simulink model "inverter_pwmDC_test"  (R2018b)
settings: Solver=ode23tb  StartTime=0.0  StopTime=10.0  RelTol=1e-3
undefined symbols (not defined in the file): Cfmax, Lf, RLf, Tss
libraries: powerlib x8, powerlib_meascontrol x4, dspsrcs4 x3, pePowerMeasurement x2, re_lib x1, simulink x1
settings Model: Creator=samuel  LastModifiedBy=samuel

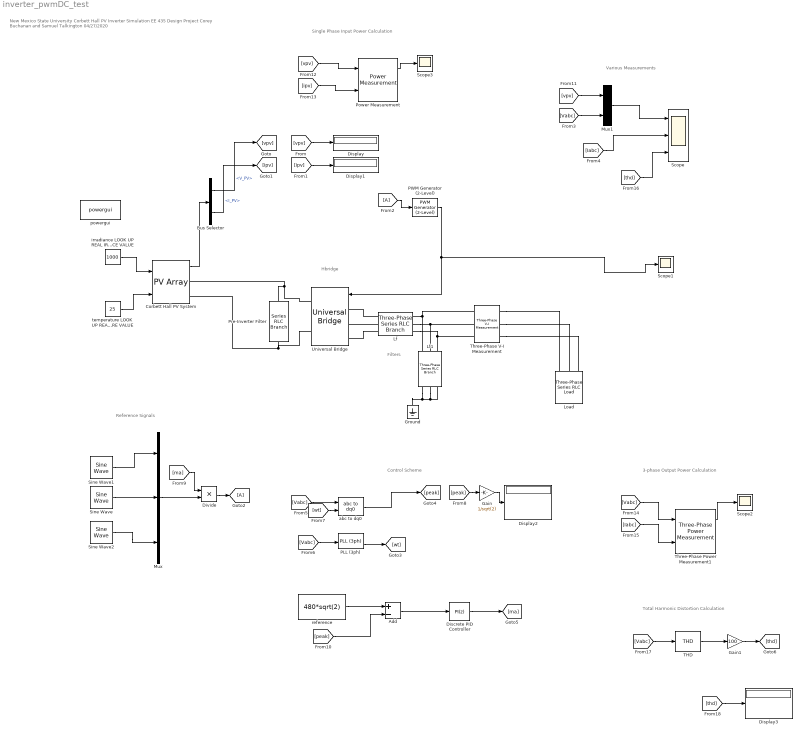
== system inverter_pwmDC_test ==
  note: Hbridge
  note: Filters
  note: Various Measurements
  note: Total Harmonic Distortion Calculation
  note: New Mexico State University Corbett Hall PV Inverter Simulation
      | EE 435 Design Project
      | Corey Buchanan and Samuel Talkington
      | 04/27/2020
  note: Control Scheme
  note: Reference Signals
  note: 3-phase Output Power Calculation
  note: Single Phase Input Power Calculation
  Add : Sum  Inputs=+-
  Bus Selector : BusSelector  OutputSignals=V_PV,I_PV
  Corbett Hall PV System : re_lib/Solar/PV Array  Npar=12  Nser=16  PlotType=array @ 1000 W/m2 & specified temperatures  S_vec="[ 1000  500  100 ]"  Temp_C_vec="[ 45 25  ]"  ModuleName=User-defined  PlotWhenSelected=off  Pm=420.28  Ncell=144  Voc=48  Isc=11.26  Vm=39.5  Im=10.64  beta_Voc_pc=-0.29  alpha_Isc_pc=0.05  beta_Voc=-0.1392  alpha_Isc=0.00563  IL=11.3192  I0=2.4941e-11  nI=0.48371  Rsh=229.1137  Rs=0.28191  BAL=on  Tc=1e-6  Tfilter=5e-5
  Discrete PID Controller : simulink/Continuous/PID Controller  Controller=PI  Form=Parallel  TimeDomain=Discrete-time  SampleTime=Tss*100  IntegratorMethod=Forward Euler  FilterMethod=Forward Euler  ControllerParametersSource=internal  P=0.001  I=0.5  D=0  UseFilter=on  N=100  TunerSelectOption=Transfer Function Based (PID Tuner App)  InitialConditionSource=internal  InitialConditionForIntegrator=0  InitialConditionForFilter=0  DifferentiatorICPrevScaledInput=0  ExternalReset=none  TrackingMode=off  Kt=1  LimitOutput=on  UpperSaturationLimit=0.95  LowerSaturationLimit=0.3  LinearizeAsGain=off  AntiWindupMode=none  Kb=1  POutMin=[]  POutMax=[]  IOutMin=[]  IOutMax=[]  DOutMin=[]  DOutMax=[]  NOutMin=[]  NOutMax=[]  SumOutMin=[]  SumOutMax=[]  SaturationOutMin=[]  SaturationOutMax=[]  PParamMin=[]  PParamMax=[]  IParamMin=[]  IParamMax=[]  DParamMin=[]  DParamMax=[]  NParamMin=[]  NParamMax=[]  KbParamMin=[]  KbParamMax=[]  KtParamMin=[]  KtParamMax=[]  KbOutMin=[]  KbOutMax=[]  KtOutMin=[]  KtOutMax=[]  IntegratorOutMin=[]  IntegratorOutMax=[]  FilterOutMin=[]  FilterOutMax=[]  SumI1OutMin=[]  SumI1OutMax=[]  SumI2OutMin=[]  SumI2OutMax=[]  SumI3OutMin=[]  SumI3OutMax=[]  SumI4OutMin=[]  SumI4OutMax=[]  SumDOutMin=[]  SumDOutMax=[]  DifferentiatorOutMin=[]  DifferentiatorOutMax=[]  FilterDiffOutCoefMin=[]  FilterDiffOutCoefMax=[]  ReciprocalOutMin=[]  ReciprocalOutMax=[]  SumDenOutMin=[]  SumDenOutMax=[]  SumNumOutMin=[]  SumNumOutMax=[]  DivideOutMin=[]  DivideOutMax=[]  IntegratorContinuousStateAttributes=''  IntegratorStateMustResolveToSignalObject=off  IntegratorRTWStateStorageClass=Auto  FilterContinuousStateAttributes=''  FilterStateMustResolveToSignalObject=off  FilterRTWStateStorageClass=Auto  ParallelPVariant=InternalParameters  IdealPVariant=Disabled  IVariant=InternalParameters  DVariant=Disabled  IntegratorVariant=Discrete  SatVariant=Enabled  AWVariant=Passthrough  PCopyVariant=Disabled  TRVariant=Disabled  FdbkBlocksVariant=Forward  IdealPFdbkVariant=Disabled  SatFdbkVariant=Disabled  DerivativeFilterVariant=Disabled  NVariant=Disabled  NCopyVariant=Disabled_SignalSpec  FilterICVariant=Disabled  IntegratorICVariant=InternalICs  ExternalResetVariant=Disabled  TRSumVariant=Passthrough  SumFdbkVariant=Disabled  SumVariant=Sum_PI
  Display{,1..3} (4 alike) : Display
  Divide : Product  Inputs=**
  Gain : Gain  Gain=1/sqrt(2)
  Gain1 : Gain  Gain=100
  Ground : powerlib/Elements/Ground  LConnTagsString=a
  Lf : powerlib/Elements/Three-Phase Series RLC Branch  LConnTagsString=A|B|C  RConnTagsString=A|B|C  BranchType=RL  Resistance=RLf  Inductance=Lf  Capacitance=1e-6  Measurements=None
  Lf1 : powerlib/Elements/Three-Phase Series RLC Branch  LConnTagsString=A|B|C  RConnTagsString=A|B|C  BranchType=RC  Resistance=1e-6  Inductance=Lf  Capacitance=Cfmax  Measurements=None
  "Load " : powerlib/Elements/Three-Phase Series RLC Load  LConnTagsString=A|B|C  Configuration=Y (grounded)  NominalVoltage=480  Vabc=[1e3 1e3 1e3]  Vabcp=[1e3 1e3 1e3]  NominalFrequency=60  UnbalancedPower=off  ActivePower=1  InductivePower=0  CapacitivePower=0  Pabc=[10e3 9e3 11e3]  QLabc=[100 90 110]  QCabc=[100 90 110]  Pabcp=[10e3 9e3 11e3]  QLabcp=[100 90 110]  QCabcp=[100 90 110]  Measurements=None  LoadType=constant Z
  Mux : Mux  Inputs=3
  Mux1 : Mux  Inputs=2
  PLL (3ph) : powerlib_meascontrol/PLL/PLL (3ph)  Fmin=45  Par_Init=[0, 60]  ParK=[180, 3200, 1]  TcD=1e-4  MaxRateChangeFreq=12  FilterCutOffFreq=25  Ts=Tss  AGC=on
  PWM Generator (2-Level) : powerlib_meascontrol/Pulse & Signal Generators/PWM Generator (2-Level)  ModulatorType=Three-phase bridge (6 pulses)  ModulatorMode=Unsynchronized  Fc=fsw  Pc=90  nF=27  MinMax="[ -1  1 ]"  SamplingTechnique=Natural  ModulatingSignals=off  m=0.8  Freq=60  Phase=0  Ts=Tss  ShowCarrierOutport=off
      settings: SourceProductName=Simscape Power Systems
  Power Measurement : pePowerMeasurement/Power Measurement  LabelModeActiveChoice=Continuous  F=60  K=[0 1 2 3]  Ts=0
  Pre-Inverter Filter : powerlib/Elements/Series RLC Branch  LConnTagsString=__new0  RConnTagsString=__new0  BranchType=RC  Resistance=1e-3  Inductance=1e-3  SetiL0=off  InitialCurrent=0  Capacitance=1000e-6  Setx0=on  InitialVoltage=1000  Measurements=None
  Scope : Scope  NumInputPorts=3
  Scope1 : Scope
  Scope2 : Scope
  Scope3 : Scope
  Sine Wave : dspsrcs4/Sine Wave  Amplitude=1  Frequency=60  Phase=-2*pi/3  SampleMode=Discrete  OutComplex=Real  CompMethod=Trigonometric fcn  TableSize=Speed  SampleTime=Tss  SamplesPerFrame=1  ResetState=Restart at time zero  OutputFrames=off  dataType=double  wordLen=16  udDataType=sfix(16)  fracBitsMode=Best precision  numFracBits=15  OutDataTypeStr=double  LastOutDataTypeStr=double
  Sine Wave1 : dspsrcs4/Sine Wave  Amplitude=1  Frequency=60  Phase=0  SampleMode=Discrete  OutComplex=Real  CompMethod=Trigonometric fcn  TableSize=Speed  SampleTime=Tss  SamplesPerFrame=1  ResetState=Restart at time zero  OutputFrames=off  dataType=double  wordLen=16  udDataType=sfix(16)  fracBitsMode=Best precision  numFracBits=15  OutDataTypeStr=double  LastOutDataTypeStr=double
  Sine Wave2 : dspsrcs4/Sine Wave  Amplitude=1  Frequency=60  Phase=2*pi/3  SampleMode=Discrete  OutComplex=Real  CompMethod=Trigonometric fcn  TableSize=Speed  SampleTime=Tss  SamplesPerFrame=1  ResetState=Restart at time zero  OutputFrames=off  dataType=double  wordLen=16  udDataType=sfix(16)  fracBitsMode=Best precision  numFracBits=15  OutDataTypeStr=double  LastOutDataTypeStr=double
  THD : powerlib_meascontrol/Measurements/THD  Freq=60  Ts=0
  Three-Phase V-I Measurement : powerlib/Measurements/Three-Phase V-I Measurement  VoltageMeasurement=phase-to-phase  SetLabelV=on  LabelV=Vabc  Vpu=off  VpuLL=off  CurrentMeasurement=yes  SetLabelI=on  LabelI=Iabc  Ipu=off  Pbase=100e6  Vbase=500e3  OutputType=Complex  PhasorSimulation=off  PSBequivalent=0
  Three-Phase Power Measurement1 : pePowerMeasurement/Three-Phase Power Measurement  LabelModeActiveChoice=Continuous  F=60  K=[0 1 2 3]  Seq=Positive  Ts=0
  Universal Bridge : powerlib/Power Electronics/Universal Bridge  Arms=3  SnubberResistance=1e5  SnubberCapacitance=inf  Device=MOSFET / Diodes  Ron=34e-3  Lon=0  ForwardVoltages="[  0  0  ]"  ForwardVoltage=0  GTOparameters=[ 10e-6 , 20e-6 ]  IGBTparameters=[ 1e-6 , 2e-6 ]  Measurements=None  Measurements_2=None  converterType=Rectifier
  abc to dq0 : powerlib_meascontrol/Transformations/abc to dq0  Alignment=90 degrees behind phase A axis
  irradiance LOOK UP REAL IRRADIANCE VALUE : Constant  Value=1000
  powergui : powerlib/powergui  Priority=1  SimulationMode=Discrete  SampleTime=Tss  frequency=60  Iterations=50  frequencyindice=0  Pbase=100e6  ErrMax=1e-4  UnitsV=kV  UnitsW=MW  buscounter=0  FunctionMessages=off  echomessages=off  EnableUseOfTLC=off  CurrentSourceSwitches=off  DisableSnubberDevices=off  DisableRonSwitches=off  DisableVfSwitches=off  DisplayEquations=off  SolverType=Tustin/Backward Euler (TBE)  Interpol=off  ExternalGateDelay=off  methode=off  Ts=100  x0status=blocks  SPID=on  SwTol=0  HookPort=off  RestoreLinks=warning  ResistiveCurrentMeasurement=off  Frange=[0:2:500]  Ylog=off  Xlog=on  ShowGrid=off  save=off  variable=ZData  structure=0  ZoomFFT=off  StartTime=0.0  cycles=1  DisplayStyle=1  fundamental=60  FreqAxis=off  MaxFrequency=1000  frequencyindicesteady=1  RmsSteady=1  display=off
  reference : Constant  Value=480*sqrt(2)
  temperature LOOK UP REAL TEMPERATURE VALUE : Constant  Value=25
  wires:
  temperature LOOK UP REAL TEMPERATURE VALUE/1 -> Corbett Hall PV System/2
  irradiance LOOK UP REAL IRRADIANCE VALUE/1 -> Corbett Hall PV System/1
  Corbett Hall PV System/1 -> Bus Selector/1
  Bus Selector/1 -> [vpv]  "<V_PV>"
  Bus Selector/2 -> [ipv]  "<I_PV>"
  [ipv] -> Display1/1
  [vpv] -> Display/1
  PWM Generator (2-Level)/1 -> Universal Bridge/1, Scope1/1
  Sine Wave/1 -> Mux/2
  Sine Wave1/1 -> Mux/1
  Sine Wave2/1 -> Mux/3
  [A] -> PWM Generator (2-Level)/1
  [Iabc] -> Scope/2
  [Vabc] -> abc to dq0/1
  [Vabc] -> PLL (3ph)/1
  [wt] -> abc to dq0/2
  PLL (3ph)/2 -> [wt]
  [peak] -> Gain/1
  Gain/1 -> Display2/1
  abc to dq0/1 -> [peak]
  Discrete PID Controller/1 -> [ma]
  Mux/1 -> Divide/2
  Divide/1 -> [A]
  [ma] -> Divide/1
  Add/1 -> Discrete PID Controller/1
  [peak] -> Add/2
  reference/1 -> Add/1
  [Vabc] -> Mux1/2
  Mux1/1 -> Scope/1
  [vpv] -> Mux1/1
  [ipv] -> Power Measurement/2
  [vpv] -> Power Measurement/1
  [Vabc] -> Three-Phase Power Measurement1/1
  [Iabc] -> Three-Phase Power Measurement1/2
  Three-Phase Power Measurement1/1 -> Scope2/1
  Power Measurement/1 -> Scope3/1
  [Vabc] -> THD/1
  THD/1 -> Gain1/1
  Gain1/1 -> [thd]
  [thd] -> Scope/3
  [thd] -> Display3/1
  connections:
  Universal Bridge/RConn1 -- Corbett Hall PV System/RConn1 -- Pre-Inverter Filter/LConn1
  Universal Bridge/RConn2 -- Corbett Hall PV System/RConn2 -- Pre-Inverter Filter/RConn1
  Lf/LConn1 -- Universal Bridge/LConn1
  Lf/LConn2 -- Universal Bridge/LConn2
  Lf/LConn3 -- Universal Bridge/LConn3
  Lf/RConn1 -- Three-Phase V-I Measurement/LConn1 -- Lf1/LConn1
  Lf/RConn2 -- Three-Phase V-I Measurement/LConn2 -- Lf1/LConn2
  Lf/RConn3 -- Three-Phase V-I Measurement/LConn3 -- Lf1/LConn3
  Lf1/RConn1 -- Lf1/RConn3 -- Lf1/RConn2 -- Ground/LConn1
  Three-Phase V-I Measurement/RConn1 -- "Load "/LConn1
  Three-Phase V-I Measurement/RConn2 -- "Load "/LConn2
  Three-Phase V-I Measurement/RConn3 -- "Load "/LConn3
